simulink model "PUIO"  (R2016b)
settings: Solver=ode45  StartTime=0.0  StopTime=10.0  RelTol=1e-3  EnableMultiTasking=on
values from neighbouring files (symbols this model uses):
  C = eye(7)    [DPUIOv2.m]    (also in DPUIOv3.m; amirsCalcs.m)
  F = A1-G1*c1    [DPUIOv2.m]    (also in DPUIOv3.m = A1 - G1*c1; amirsCalcs.m = A1 - G1*C)
  f1Val = 10    [DPUIOv2.m]    (also in DPUIOv3.m)
  f2Val = 10    [DPUIOv2.m]    (also in DPUIOv3.m)
  f3Val = 10    [DPUIOv2.m]    (also in DPUIOv3.m)
  f4Val = 10    [DPUIOv2.m]    (also in DPUIOv3.m)
  f5Val = 10    [DPUIOv2.m]    (also in DPUIOv3.m)
  f6Val = 10    [DPUIOv2.m]    (also in DPUIOv3.m)
  f7Val = 10    [DPUIOv2.m]    (also in DPUIOv3.m)
  flt1 = 0    [DPUIOv2.m]    (also in DPUIOv3.m)
  flt2 = 1    [DPUIOv2.m]    (also in DPUIOv3.m)
  flt3 = 0    [DPUIOv2.m]    (also in DPUIOv3.m)
  flt4 = 0    [DPUIOv2.m]    (also in DPUIOv3.m)
  flt5 = 0    [DPUIOv2.m]    (also in DPUIOv3.m)
  flt6 = 0    [DPUIOv2.m]    (also in DPUIOv3.m)
  flt7 = 0    [DPUIOv2.m]    (also in DPUIOv3.m)
  L = Deg-Ag    [DPUIOv2.m]    (also in DPUIOv3.m; amirsCalcs.m)
  N = E*CEg    [DPUIOv2.m]    (also in DPUIOv3.m; amirsCalcs.m = Ed* pinv(C*Ed))
  tf1 = 2    [DPUIOv2.m]    (also in DPUIOv3.m)
  tf2 = 2    [DPUIOv2.m]    (also in DPUIOv3.m)
  tf3 = 2    [DPUIOv2.m]    (also in DPUIOv3.m)
  tf4 = 2    [DPUIOv2.m]    (also in DPUIOv3.m)
  tf5 = 2    [DPUIOv2.m]    (also in DPUIOv3.m)
  tf6 = 5    [DPUIOv2.m]    (also in DPUIOv3.m)
  tf7 = 7    [DPUIOv2.m]    (also in DPUIOv3.m)
  x0 = [0 1 1 0 0 0 0]    [DPUIOv2.m]    (also in DPUIOv3.m; amirsCalcs.m)
settings Model: Creator=sqn4594  LastModifiedBy=samnazari
settings DataIOCC: LimitDataPoints=on  SaveFormat=Array
settings OptimizationCC: LifeSpan=inf
settings DebuggingCC: SolverPrmCheckMsg=warning  FcnCallInpInsideContextMsg=warning  AllowSymbolicDim=off  SFUnexpectedBacktrackingDiag=warning  SFNoUnconditionalDefaultTransitionDiag=warning  SFExecutionAtInitializationDiag=none
settings HardwareCC: ProdBitPerPointer=32  ProdBitPerSizeT=32  ProdBitPerPtrDiffT=32  ProdLargestAtomicFloat=None  ProdIntDivRoundTo=Undefined  ProdEndianess=Unspecified  ProdWordSize=32  ProdHWDeviceType=32-bit Generic
settings ModelReferenceCC: PropagateSignalLabelsOutOfModel=off
settings GRTTargetCC: TargetLangStandard=C89/C90 (ANSI)  GeneratePreprocessorConditionals=Disable all
settings ConfigComp: CovMetricSettings=dw  CovHtmlReporting=on  CovSaveCumulativeToWorkspaceVar=on  CovSaveSingleToWorkspaceVar=on  CovExternalEMLEnable=off

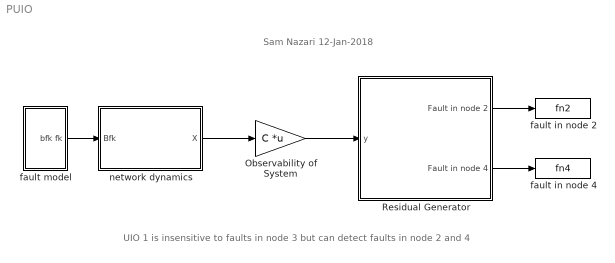
== system PUIO ==
  note: UIO 1 is insensitive to faults in node 3 but can detect faults in node 2 and 4
  note: Sam Nazari
      | 12-Jan-2018
  Observability of System : Gain  Gain=C  Multiplication=Matrix(K*u)
  Residual Generator : Subsystem
  fault model : Subsystem
  fault in node 2 : ToWorkspace  VariableName=fn2  SaveFormat=Timeseries  SampleTime=-1
  fault in node 4 : ToWorkspace  VariableName=fn4  SaveFormat=Timeseries  SampleTime=-1
  network dynamics : Subsystem
  wires:
  fault model/1(bfk fk) -> network dynamics/1(Bfk)
  network dynamics/1(X) -> Observability of System/1
  Observability of System/1 -> Residual Generator/1(y)
  Residual Generator/1(Fault in node 2) -> fault in node 2/1
  Residual Generator/2(Fault in node 4) -> fault in node 4/1

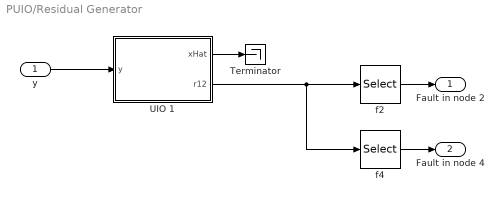
== system PUIO/Residual Generator ==
  y : Inport
  Terminator : Terminator
  UIO 1 : Subsystem
  f2 : Selector  InputPortWidth=7  IndexOptions=Index vector (dialog)  Indices=2  OutputSizes=1
  f4 : Selector  InputPortWidth=7  IndexOptions=Index vector (dialog)  Indices=4  OutputSizes=1
  Fault in node 2 : Outport
  Fault in node 4 : Outport  Port=2
  wires:
  UIO 1/1("xHat ") -> Terminator/1
  UIO 1/2(r12) -> f4/1, f2/1
  y/1 -> UIO 1/1(y)
  f2/1 -> Fault in node 2/1
  f4/1 -> Fault in node 4/1

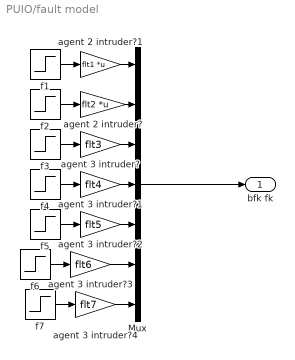
== system PUIO/fault model ==
  Mux : Mux  Inputs=7
  agent 2 intruder? : Gain  Gain=flt2  Multiplication=Matrix(K*u)
  agent 2 intruder?1 : Gain  Gain=flt1  Multiplication=Matrix(K*u)
  agent 3 intruder? : Gain  Gain=flt3
  agent 3 intruder?1 : Gain  Gain=flt4
  agent 3 intruder?2 : Gain  Gain=flt5
  agent 3 intruder?3 : Gain  Gain=flt6
  agent 3 intruder?4 : Gain  Gain=flt7
  f1 : Step  After=f1Val  SampleTime=tf1
  f2 : Step  After=f2Val  SampleTime=tf2
  f3 : Step  After=f3Val  SampleTime=tf3
  f4 : Step  After=f4Val  SampleTime=tf4
  f5 : Step  After=f5Val  SampleTime=tf5
  f6 : Step  After=f6Val  SampleTime=tf6
  f7 : Step  After=f7Val  SampleTime=tf7
  bfk fk : Outport
  wires:
  Mux/1 -> bfk fk/1
  f1/1 -> agent 2 intruder?1/1
  f2/1 -> agent 2 intruder?/1
  f3/1 -> agent 3 intruder?/1
  agent 2 intruder?/1 -> Mux/2
  agent 3 intruder?/1 -> Mux/3
  agent 2 intruder?1/1 -> Mux/1
  f4/1 -> agent 3 intruder?1/1
  agent 3 intruder?1/1 -> Mux/4
  agent 3 intruder?2/1 -> Mux/5
  f5/1 -> agent 3 intruder?2/1
  f6/1 -> agent 3 intruder?3/1
  agent 3 intruder?3/1 -> Mux/6
  f7/1 -> agent 3 intruder?4/1
  agent 3 intruder?4/1 -> Mux/7

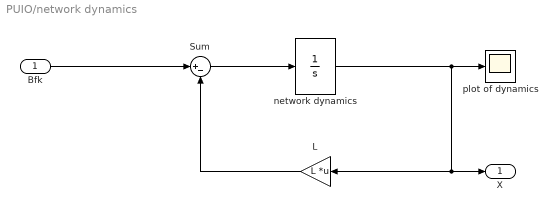
== system PUIO/network dynamics ==
  Bfk : Inport
  L : Gain  Gain=L  Multiplication=Matrix(K*u)
  Sum : Sum  Inputs=|+-
  network dynamics : Integrator  InitialCondition=x0
  plot of dynamics : Scope
  X : Outport
  wires:
  Bfk/1 -> Sum/1
  Sum/1 -> network dynamics/1
  network dynamics/1 -> plot of dynamics/1, X/1, L/1
  L/1 -> Sum/2

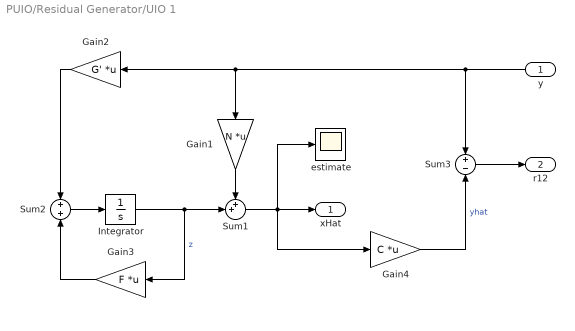
== system PUIO/Residual Generator/UIO 1 ==
  y : Inport
  Gain1 : Gain  Gain=N  Multiplication=Matrix(K*u)
  Gain2 : Gain  Gain=G'  Multiplication=Matrix(K*u)
  Gain3 : Gain  Gain=F  Multiplication=Matrix(K*u)
  Gain4 : Gain  Gain=C  Multiplication=Matrix(K*u)
  Integrator : Integrator  InitialCondition=x0
  Sum1 : Sum  Inputs=++|
  Sum2 : Sum
  Sum3 : Sum  Inputs=+-
  estimate : Scope
  "xHat " : Outport
  r12 : Outport  Port=2
  wires:
  Sum2/1 -> Integrator/1
  Integrator/1 -> Sum1/2, Gain3/1  "z"
  Gain2/1 -> Sum2/1
  Gain3/1 -> Sum2/2
  Gain1/1 -> Sum1/1
  Sum1/1 -> Gain4/1, estimate/1, "xHat "/1
  Gain4/1 -> Sum3/2  "yhat"
  Sum3/1 -> r12/1
  y/1 -> Sum3/1, Gain1/1, Gain2/1
